simulink model "thyristor_three_phase_ac_converter"  (R2023b)
settings: Solver=VariableStepAuto  StartTime=0.0  StopTime=2.0  RelTol=1e-3
libraries: spsThyristorLib x6, spsVoltageMeasurementLib x4, spsCurrentMeasurementLib x2, spsSeriesRLCBranchLib x1, spsThreePhaseSourceLib x1, sps_lib x1
settings Model: Creator=nandhitha  LastModifiedBy=essa7

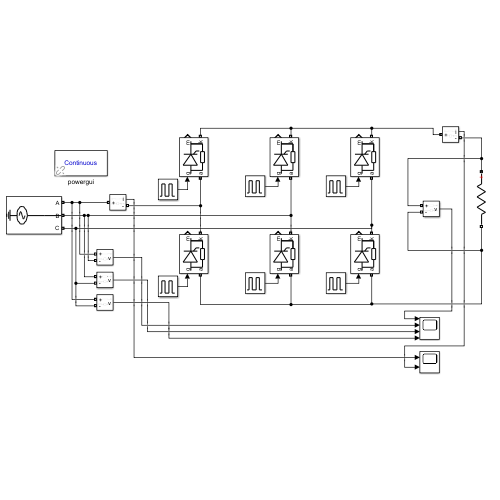
[thumbnail: Simulink's stored preview of the top-level diagram]
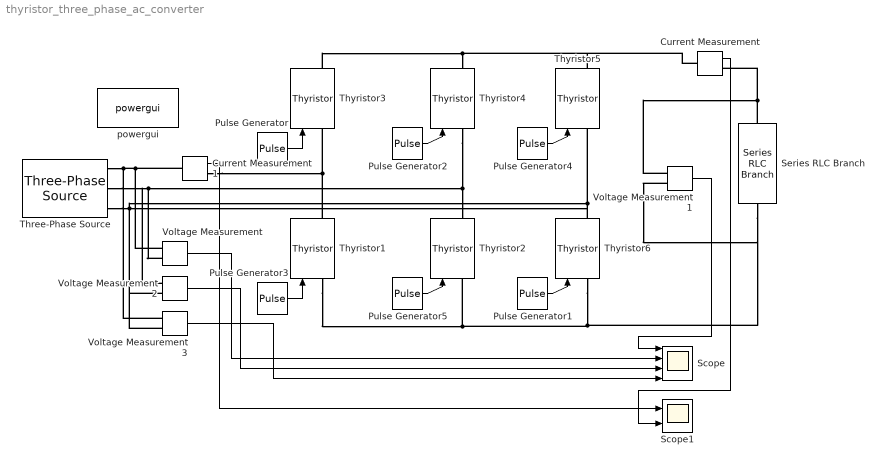
== system thyristor_three_phase_ac_converter ==
  Current Measurement : spsCurrentMeasurementLib/Current Measurement  PhasorSimulation=off  OutputType=Complex  PSBequivalent=0
  Current Measurement1 : spsCurrentMeasurementLib/Current Measurement  PhasorSimulation=off  OutputType=Complex  PSBequivalent=0
  Pulse Generator : DiscretePulseGenerator  PulseType=Time based  Amplitude=230  Period=0.02  PulseWidth=10  PhaseDelay=30*0.02/360
  Pulse Generator1 : DiscretePulseGenerator  PulseType=Time based  Amplitude=230  Period=0.02  PulseWidth=10  PhaseDelay=(30+60)*0.02/360
  Pulse Generator2 : DiscretePulseGenerator  PulseType=Time based  Amplitude=230  Period=0.02  PulseWidth=10  PhaseDelay=(30+120)*0.02/360
  Pulse Generator3 : DiscretePulseGenerator  PulseType=Time based  Amplitude=230  Period=0.02  PulseWidth=10  PhaseDelay=(30+180)*0.02/360
  Pulse Generator4 : DiscretePulseGenerator  PulseType=Time based  Amplitude=230  Period=0.02  PulseWidth=10  PhaseDelay=(30+240)*0.02/360
  Pulse Generator5 : DiscretePulseGenerator  PulseType=Time based  Amplitude=230  Period=0.02  PulseWidth=10  PhaseDelay=(30+300)*0.02/360
  Scope : Scope  NumInputPorts=4
  Scope1 : Scope  NumInputPorts=2
  Series RLC Branch : spsSeriesRLCBranchLib/Series RLC Branch  LConnTagsString=__new0  RConnTagsString=__new0  BranchType=R  Resistance=2  Inductance=1e-3  SetiL0=off  InitialCurrent=0  Capacitance=1e-6  Setx0=off  InitialVoltage=0  Measurements=None
  Three-Phase Source : spsThreePhaseSourceLib/Three-Phase Source  InternalConnection=Yg  VoltagePhases=off  Voltage=230  PhaseAngle=0  Voltage_phases=[25e3 25e3 25e3]/sqrt(3)  PhaseAngles_phases=[0 -120 +120]  Frequency=50  NonIdealSource=off  SpecifyImpedance=off  Resistance=0.8929  Inductance=16.58e-3  ShortCircuitLevel=100e6  BaseVoltage=400  XRratio=7  BusType=swing  Pref=10e3  Qref=0  Prefabc=[10e3, 10e3, 10e3]  Qrefabc=[0, 0, 0]  Qmin=-inf  Qmax=inf
  Thyristor{1..6} (6 alike) : spsThyristorLib/Thyristor  Ron=0.001  Lon=0  Vf=0.8  IC=0  Rs=500  Cs=250e-9  Measurements=on
  Voltage Measurement{,1..3} (4 alike) : spsVoltageMeasurementLib/Voltage Measurement  PhasorSimulation=off  OutputType=Complex  PSBequivalent=0
  powergui : sps_lib/powergui  Priority=1  SimulationMode=Continuous  SampleTime=50e-6  frequency=60  Iterations=50  frequencyindice=50  Pbase=100e6  ErrMax=1e-4  UnitsV=kV  UnitsW=MW  buscounter=0  FunctionMessages=off  echomessages=off  EnableUseOfTLC=off  CurrentSourceSwitches=off  DisableSnubberDevices=off  DisableRonSwitches=off  DisableVfSwitches=off  DisplayEquations=off  AutomaticDiscreteSolvers=off  SolverType=Tustin/Backward Euler (TBE)  Interpol=off  ExternalGateDelay=off  methode=off  Ts=100  x0status=blocks  SPID=on  SwTol=0  HookPort=off  NonlinearTolerance=1e-4  nMaxIteration=100  ContinueOnMaxIteration=off  RestoreLinks=warning  ResistiveCurrentMeasurement=off  Frange=[0:2:500]  Ylog=off  Xlog=on  ShowGrid=off  save=off  variable=ZData  structure=0  ZoomFFT=off  StartTime=0.0  cycles=1  DisplayStyle=1  fundamental=60  FreqAxis=off  MaxFrequency=1000  frequencyindicesteady=1  RmsSteady=1  display=off
  wires:
  Voltage Measurement1/1 -> Scope/1
  Voltage Measurement/1 -> Scope/2
  Current Measurement/1 -> Scope1/2
  Voltage Measurement2/1 -> Scope/3
  Voltage Measurement3/1 -> Scope/4
  Pulse Generator/1 -> Thyristor3/1
  Pulse Generator1/1 -> Thyristor6/1
  Pulse Generator2/1 -> Thyristor4/1
  Pulse Generator3/1 -> Thyristor1/1
  Pulse Generator4/1 -> Thyristor5/1
  Pulse Generator5/1 -> Thyristor2/1
  Current Measurement1/1 -> Scope1/1
  connections:
  Voltage Measurement/LConn1 -- Current Measurement1/LConn1 -- Voltage Measurement3/LConn1 -- Three-Phase Source/RConn1
  Thyristor1/LConn1 -- Voltage Measurement1/LConn2 -- Series RLC Branch/RConn1 -- Thyristor6/LConn1 -- Thyristor2/LConn1
  Thyristor3/RConn1 -- Current Measurement/LConn1 -- Thyristor5/RConn1 -- Thyristor4/RConn1
  Thyristor4/LConn1 -- Voltage Measurement2/LConn1 -- Three-Phase Source/RConn2 -- Voltage Measurement/LConn2 -- Thyristor2/RConn1
  Thyristor6/RConn1 -- Voltage Measurement3/LConn2 -- Voltage Measurement2/LConn2 -- Three-Phase Source/RConn3 -- Thyristor5/LConn1
  Series RLC Branch/LConn1 -- Voltage Measurement1/LConn1 -- Current Measurement/RConn1
  Thyristor1/RConn1 -- Current Measurement1/RConn1 -- Thyristor3/LConn1
